simulink model "Prova_1_HDLtest"  (R2023b)
settings: Solver=FixedStepAuto  StartTime=0.0  StopTime=10  FixedStep=0.01  RelTol=1e-3  EnableMultiTasking=on
model workspace (MAT data in the model file):
  socvcb = containers.Map
  socvcb.serialization.keys = {15.0001220703, 41.0002441406, 17209.0001221, 24395.0008545}
  socvcb.serialization.values : function handle (value not decoded)
  socvcb.serialization.uniformity = 0
  socvcb.serialization.keyType = 'double'
  socvcb.serialization.valueType = 'any'
libraries: prociolib x3, hwlogicconnlib x2, socmemlib x2, proctasklib x1
settings Model: Creator=lenovo GAME  LastModifiedBy=lenovo GAME
settings SolverCC: PositivePriorityOrder=on
settings OptimizationCC: EnhancedBackFolding=on  PassReuseOutputArgsAs=Individual arguments  ZeroExternalMemoryAtStartup=off  ZeroInternalMemoryAtStartup=off  MaxStackSize=64  OptimizeBlockOrder=speed  DifferentSizesBufferReuse=on  OptimizationCustomize=off  EfficientTunableParamExpr=on
settings DebuggingCC: ParameterTunabilityLossMsg=error
settings HardwareCC: ProdBitPerPointer=32  ProdBitPerSizeT=32  ProdBitPerPtrDiffT=32  ProdLargestAtomicFloat=None  ProdWordSize=32  ProdHWDeviceType=Custom Processor->Custom  HardwareBoardFeatureSet=SoCBlockset
settings ModelReferenceCC: ModelReferenceNumInstancesAllowed=Single
settings SFSimCC: MATLABDynamicMemAlloc=off
settings RTWCC: Description=Embedded Coder  SystemTargetFile=ert.tlc  HardwareBoard=Custom Hardware Board  TLCOptions="-aInlineSetEventsForThisBaseRateFcn=TLC_FALSE -aSuppressMultiTaskScheduler=TLC_FALSE  -aRateBasedStepFcn=0"  TemplateMakefile=ert_default_tmf
settings CodeAppCC: ForceParamTrailComments=on  IgnoreCustomStorageClasses=off  OperatorAnnotations=on  SimulinkDataObjDesc=on  SFDataObjDesc=on  InsertBlockDesc=on

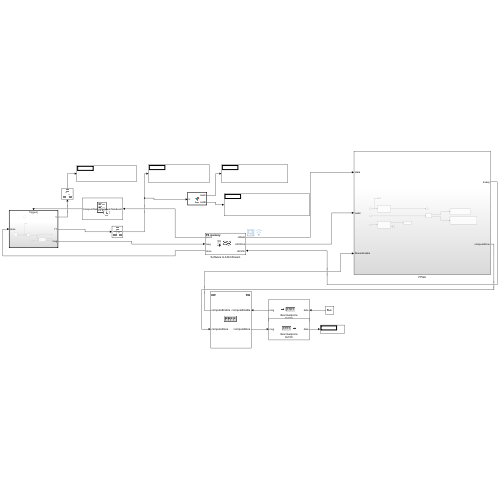
[thumbnail: Simulink's stored preview of the top-level diagram]
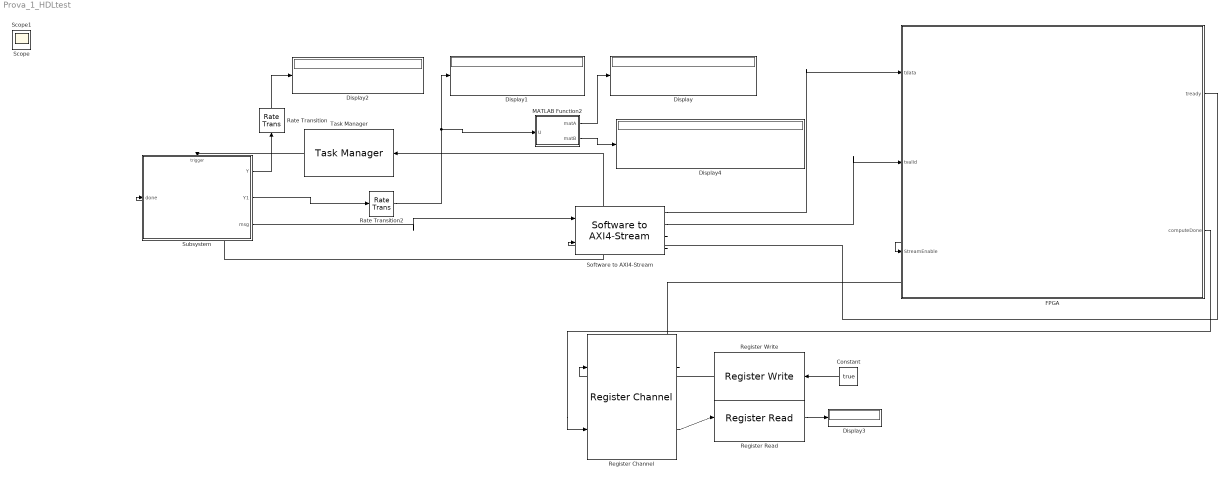
== system Prova_1_HDLtest ==
  Constant : Constant  Value=true
  Display{,1..4} (5 alike) : Display
  FPGA : Subsystem
  MATLAB Function2 : MATLAB Function  TreatAsAtomicUnit=on
  Rate Transition : RateTransition  Deterministic=off
  Rate Transition2 : RateTransition  Deterministic=off
  Register Channel : socmemlib/Register Channel  RegisterTable={ 'computeEnable', 'Write', 'boolean', '1'; 'computeDone', 'Read', 'uint32', '1' }  SampleTime=-1  RegTableNames={'computeEnable' 'computeDone' }  RegTableRW={'Write' 'Read' }  RegTableDataTypes={'boolean' 'uint32' }  RegTableVectorSizes={'1' '1' }  NumRegisters=2  RegTableDefaultValues="{'x\"0000\"' 'x\"0000\"' }"  RegTableDirty=0
  Register Read : prociolib/Register Read  DeviceName=/dev/mwipcore  OffsetAddress=hex2dec('0100')  OutDataTypeStr=boolean  OutputVectorSize=1  SampleTime=-1  Dummy=0
  Register Write : prociolib/Register Write  OutputSink=To output port  TunableParamName=A  RegisterName=RegA  DeviceName=/dev/mwipcore  OffsetAddress=hex2dec('100')  Dummy=0
  Software to AXI4-Stream : socmemlib/Software to AXI4-Stream  MemorySimulation=Burst accurate  MemorySelection=PS memory  MRNumBuffers=8  BurstLengthReaderChIf=25  FIFODepthReader=8  FIFOAFullDepthReader=6  ICClockFrequencyReader=100  ICDataWidthReader=64  ChDimensionsWriterChIf=25  ChTypeWriterChIf=uint64  ChDimensionsReaderChIf=25  ChTypeReaderChIf=double  ChFrameSampleTimeReaderChIf=1  ChBitPackedReaderChIf=off  LastTargetBoard=Custom Hardware Board  MRRegionSize=1600  MRBufferSize=200  DiagnosticLevel=No debug
  Subsystem : Subsystem
  Task Manager : proctasklib/Task Manager  AllTaskData="{\"taskName\":\"ComputeTask\",\"taskType\":\"Event-driven\",\"taskEvent\":\"ComputeTaskEvent\",\"taskPeriod\":\"0.1\",\"taskPriority\":\"50\",\"coreSelection\":\"Specified core\",\"coreNum\":\"0\",\"dropOverranTasks\":false,\"playbackRecorded\":false,\"diagnosticsFile\":\"\",\"taskDurationSource\":\"Dialog\",\"taskDuration\":1E-6,\"taskDurationDeviation\":0,\"logExecutionData\":true,\"logDroppedTasks\":false,\"version\":\"2.6\",\"taskDurationData\":{\"percent\":\"100\",\"mean\":\"1e-06\",\"dev\":\"0\",\"min\":\"1e-06\",\"max\":\"1e-06\"},\"taskEventSource\":\"Unspecified\",\"taskEventSourceAssignmentType\":\"Unassigned\",\"taskEventSourceType\":\"Unspecified\",\"taskEventGroup\":\"Unspecified\",\"taskEventInterrupt\":\"Unspecified\",\"taskEventOrder\":1,\"taskDisablePremption\":false,\"taskClearInterruptFlagsAtEndOfEvent\":false}"  EnableTaskSimulation=on  StreamToSDI=on  WriteToFile=off  OverwriteFile=off  SupportEventPorts=on  UseScheduleEditor=off  CustomizationInfo=''
  Scope : Scope
  Scope1 : Scope
  wires:
  MATLAB Function2/1(matA) -> Display/1
  Subsystem/2(Y1) -> Rate Transition2/1
  Subsystem/1(Y) -> Rate Transition/1
  Software to AXI4-Stream/3 -> Task Manager/1
  Task Manager/1 -> Subsystem/Trigger
  Software to AXI4-Stream/4 -> Subsystem/1(done)
  Subsystem/3(msg) -> Software to AXI4-Stream/1
  Rate Transition2/1 -> MATLAB Function2/1(U), Display1/1
  Rate Transition/1 -> Display2/1
  Software to AXI4-Stream/1 -> FPGA/1(tdata)
  Software to AXI4-Stream/2 -> FPGA/2(tvalid)
  FPGA/1(tready) -> Software to AXI4-Stream/2
  Register Channel/1 -> FPGA/3(StreamEnable)
  Constant/1 -> Register Write/1
  FPGA/2(computeDone) -> Register Channel/2
  Register Channel/2 -> Register Read/1
  Register Read/1 -> Display3/1
  Register Write/1 -> Register Channel/1
  MATLAB Function2/2(matB) -> Display4/1

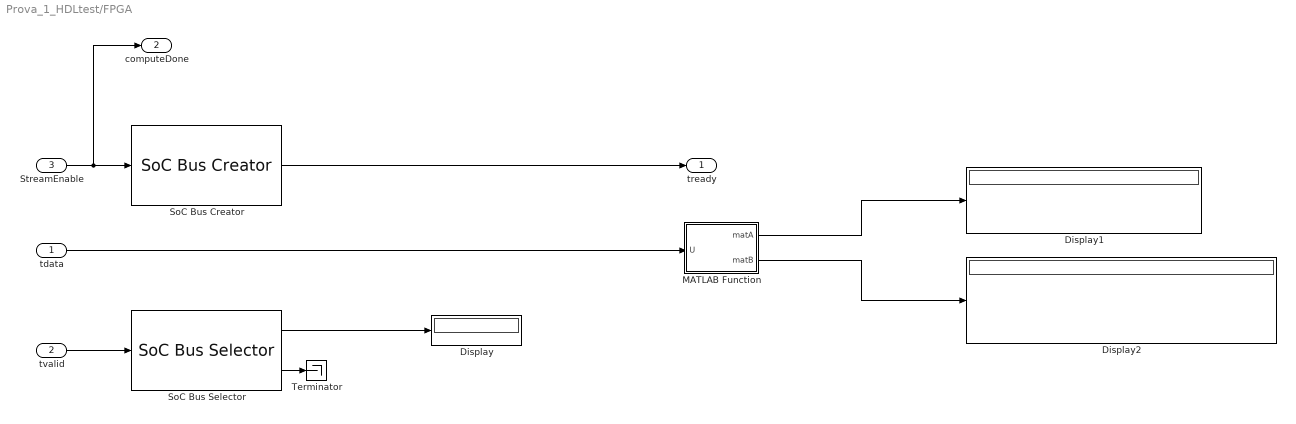
== system Prova_1_HDLtest/FPGA ==
  tdata : Inport
  tvalid : Inport  Port=2
  StreamEnable : Inport  Port=3
  Display : Display
  Display1 : Display
  Display2 : Display
  MATLAB Function : MATLAB Function  TreatAsAtomicUnit=on
  SoC Bus Creator : hwlogicconnlib/SoC Bus Creator  Protocol=Data stream  ctrltype=Ready
  SoC Bus Selector : hwlogicconnlib/SoC Bus Selector  Protocol=Data stream  ctrltype=Valid
  Terminator : Terminator
  tready : Outport
  computeDone : Outport  Port=2
  wires:
  tvalid/1 -> SoC Bus Selector/1
  SoC Bus Selector/2 -> Terminator/1
  SoC Bus Selector/1 -> Display/1
  StreamEnable/1 -> computeDone/1, SoC Bus Creator/1
  SoC Bus Creator/1 -> tready/1
  tdata/1 -> MATLAB Function/1(U)
  MATLAB Function/2(matB) -> Display2/1
  MATLAB Function/1(matA) -> Display1/1

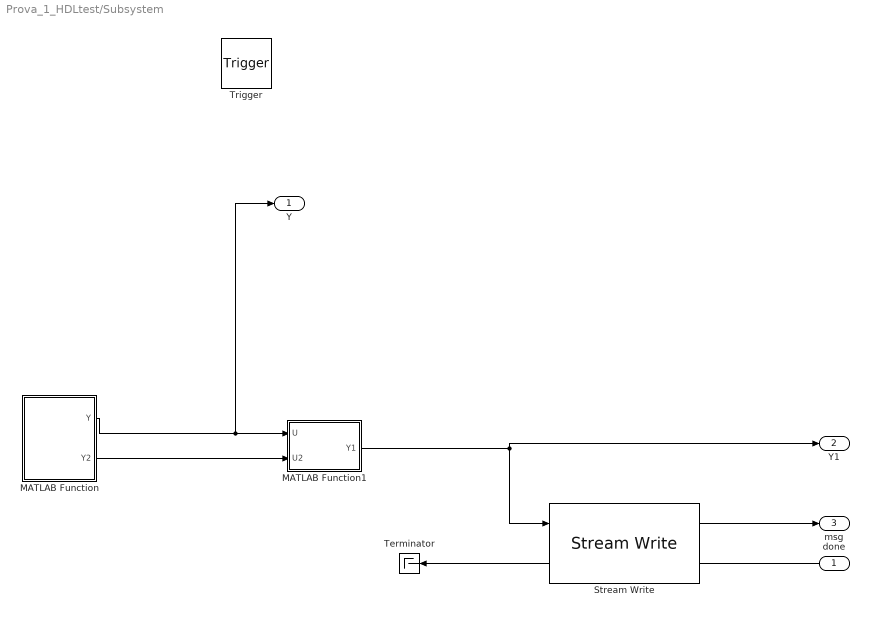
== system Prova_1_HDLtest/Subsystem ==
  done : Inport
  Trigger : TriggerPort  TriggerType=function-call  VariantControl=(inherit)  PortDimensions=1
  MATLAB Function : MATLAB Function  TreatAsAtomicUnit=on
  MATLAB Function1 : MATLAB Function  TreatAsAtomicUnit=on
  Stream Write : prociolib/Stream Write  DeviceName=ip:mm2s  NumberOfBuffers=8  EnableEvent=on
  Terminator : Terminator
  Y : Outport
  Y1 : Outport  Port=2
  msg : Outport  Port=3
  wires:
  MATLAB Function/1(Y) -> Y/1, MATLAB Function1/1(U)
  MATLAB Function1/1(Y1) -> Y1/1, Stream Write/1
  done/1 -> Stream Write/2
  Stream Write/2 -> Terminator/1
  Stream Write/1 -> msg/1
  MATLAB Function/2(Y2) -> MATLAB Function1/2(U2)

== matlab function Prova_1_HDLtest/Subsystem/MATLAB Function ==
  data: Y output; Y2 output
function [Y,Y2] = fcn()
    A = [1 2 3; 4 5 6; 7 8 9];
    B = [9 8 7; 6 5 4; 3 2 1];
    Y = A * B;
    
    C = [1 2 3 4; 5 6 7 8; 9 10 11 12; 13 14 15 16];          % o due 4x4 a piacere moltiplicate tra loro
    D = eye(4);
    Y2 = C*D;  

end

== matlab function Prova_1_HDLtest/MATLAB Function2 ==
  data: U input; matA output; matB output
function [matA, matB] = fcn(U)   % U è 25x1 double
matA = reshape(typecast(U(1:9),'double'), [3 3]);
matB = reshape(typecast(U(10:25),'double'), [4 4]);

end

== matlab function Prova_1_HDLtest/FPGA/MATLAB Function ==
  data: U input; matA output; matB output
function [matA, matB] = fcn(U)   % U è 25x1 double
matA = reshape(U(1:9), [3 3]);
matB = reshape(U(10:25), [4 4]);
end

== matlab function Prova_1_HDLtest/Subsystem/MATLAB Function1 ==
  data: U input; Y1 output; U2 input
function Y1 = fcn(U, U2)
Y1 = [typecast(U(:),'uint64'); typecast(U2(:),'uint64')];   % 9+16 = 25 elementi
end
